simulink model "two_turtlebot3_waffle_pi_modelbaseMRAC2020"  (R2020b)
settings: Solver=VariableStepAuto  StartTime=0.0  StopTime=50  FixedStep=0.0001  RelTol=1e-3
values from neighbouring files (symbols this model uses):
  m = 5    [Traj.mat]    (also in dynamic_model.m = mc+2*mw; eightshape.mat)
  w = 0.015    [Assy_StateFlow_DataFile.m]    (also in eightshape.mat)
undefined symbols (not defined in the file or in its folder): X, Y, Z
libraries: sm_lib x258, nesl_utility x21, simulink x2, robotcorelib x2
(part 5 of 5)

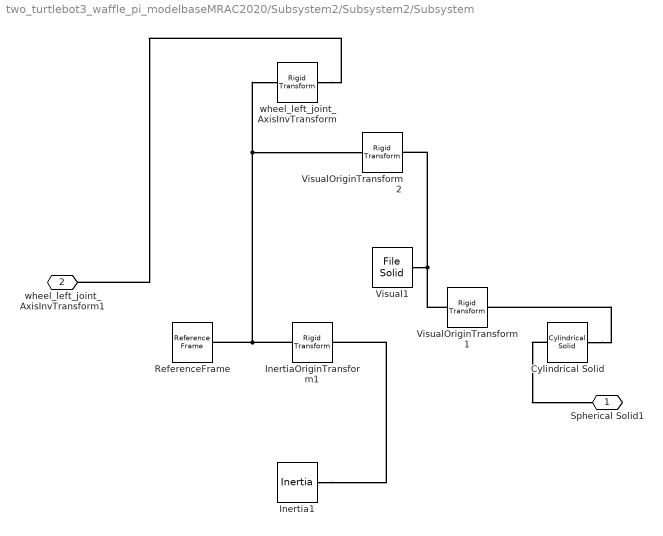
== system two_turtlebot3_waffle_pi_modelbaseMRAC2020/Subsystem2/Subsystem2/Subsystem ==
  Cylindrical Solid : sm_lib/Body Elements/Cylindrical Solid  GraphicAmbientColor=[0.15 0.15 0.15 1.0]  BasedOnType=Density  CenterOfMass=[0 0 0]  CenterOfMassUnits=m  GraphicDiffuseColor=[0.5 0.5 0.5]  CylinderLength=0.01  CylinderLengthUnits=m  CylinderRadius=0.033  CylinderRadiusUnits=m  Density=1000  DensityUnits=kg/m^3  DoExposeReferenceFrame=on  GraphicEmissiveColor=[0.0 0.0 0.0 1.0]  ExportEntireGeometry=on  SerializedFrames=<Frames/>  MarkerShape=Sphere  MarkerSize=10  GraphicType=FromGeometry  InertiaType=PointMass  Mass=0  MassUnits=kg  MomentsOfInertia=[1 1 1]  MomentsOfInertiaUnits=kg*m^2  GraphicOpacity=1.0  ProductsOfInertia=[0 0 0]  ProductsOfInertiaUnits=kg*m^2  GraphicShininess=75  GraphicSpecularColor=[0.5 0.5 0.5 1.0]  GraphicVisPropType=SimpleVisualProperties
  Inertia1 : sm_lib/Body Elements/Inertia  InertiaType=Custom  Mass=0.02849894  MassUnits=kg  CenterOfMass=[0, 0, 0]  CenterOfMassUnits=m  MomentsOfInertia=[1.117558e-05, 1.1192413e-05, 2.0712558e-05]  MomentsOfInertiaUnits=kg*m^2  ProductsOfInertia=[-1.4400107e-11, -5.9381719e-09, -4.2369783e-11]  ProductsOfInertiaUnits=kg*m^2  GraphicType=None  MarkerShape=Inertia  MarkerSize=20  GraphicVisPropType=SimpleVisualProperties  GraphicDiffuseColor=[0.5 0.5 0.5]  GraphicSpecularColor=[0.5 0.5 0.5 1.0]  GraphicAmbientColor=[0.15 0.15 0.15 1.0]  GraphicEmissiveColor=[0.0 0.0 0.0 1.0]  GraphicShininess=75  GraphicOpacity=1.0
  InertiaOriginTransform1 : sm_lib/Frames and Transforms/Rigid Transform  TranslationMethod=Cartesian  TranslationStandardOffset=0  TranslationLengthUnit=m  TranslationStandardAxis=+Z  TranslationCartesianOffset=[0, 0, 0]  TranslationROffset=0  TranslationROffsetUnits=m  TranslationZOffset=0  TranslationZOffsetUnits=m  TranslationThetaOffset=0  TranslationThetaOffsetUnits=deg  RotationMethod=RotationSequence  RotationAngleUnits=deg  RotationStandardAxis=+Z  RotationAngle=0.0  RotationArbitraryAxis=[0 0 1]  FollAlignAxisA=+X  BaseAlignAxisA=+Y  FollAlignAxisB=+Y  BaseAlignAxisB=+Z  RotationSequenceAxes=BaseAxes  RotationSequence=XYZ  RotationSequenceAngles=[0, 0, 0]  RotationSequenceAnglesUnits=rad  RotationMatrix=[1 0 0; 0 1 0; 0 0 1]
  ReferenceFrame : sm_lib/Frames and Transforms/Reference Frame
  Visual1 : sm_lib/Body Elements/File Solid  ExtGeomFileName=C:\Users\suyao\Desktop\tethered robot planning\simulation\Stateflow_Lab\CAD\right_tire.stl  UnitType=Custom  ExtGeomFileUnits=mm  StepReaderType=HEX  ExportConvexHullGeometry=on  InertiaType=Custom  Mass=0  MassUnits=kg  CenterOfMass=[0, 0, 0]  CenterOfMassUnits=m  MomentsOfInertia=[0, 0, 0]  MomentsOfInertiaUnits=kg*m^2  ProductsOfInertia=[0, 0, 0]  ProductsOfInertiaUnits=kg*m^2  BasedOnType=DensityFromFile  Density=1000  DensityUnits=kg/m^3  DoExposeReferenceFrame=on  SerializedFrames=<Frames/>  GraphicType=FromGeometry  MarkerShape=Sphere  MarkerSize=10  GraphicVisPropType=SimpleVisualProperties  GraphicDiffuseColor=[0.5, 0.5, 0.5]  GraphicSpecularColor=[0.5 0.5 0.5 1.0]  GraphicAmbientColor=[0.15 0.15 0.15 1.0]  GraphicEmissiveColor=[0.0 0.0 0.0 1.0]  GraphicShininess=75  GraphicOpacity=1
  VisualOriginTransform1 : sm_lib/Frames and Transforms/Rigid Transform  TranslationMethod=Cartesian  TranslationStandardOffset=0  TranslationLengthUnit=m  TranslationStandardAxis=+Z  TranslationCartesianOffset=[0, 0, 0]  TranslationROffset=0  TranslationROffsetUnits=m  TranslationZOffset=0  TranslationZOffsetUnits=m  TranslationThetaOffset=0  TranslationThetaOffsetUnits=deg  RotationMethod=StandardAxis  RotationAngleUnits=deg  RotationStandardAxis=+X  RotationAngle=90  RotationArbitraryAxis=[0 0 1]  FollAlignAxisA=+X  BaseAlignAxisA=+Y  FollAlignAxisB=+Y  BaseAlignAxisB=+Z  RotationSequenceAxes=BaseAxes  RotationSequence=XYZ  RotationSequenceAngles=[1.57, 0, 0]  RotationSequenceAnglesUnits=rad  RotationMatrix=[1 0 0; 0 1 0; 0 0 1]
  VisualOriginTransform2 : sm_lib/Frames and Transforms/Rigid Transform  TranslationMethod=Cartesian  TranslationStandardOffset=0  TranslationLengthUnit=m  TranslationStandardAxis=+Z  TranslationCartesianOffset=[0, 0, 0]  TranslationROffset=0  TranslationROffsetUnits=m  TranslationZOffset=0  TranslationZOffsetUnits=m  TranslationThetaOffset=0  TranslationThetaOffsetUnits=deg  RotationMethod=RotationSequence  RotationAngleUnits=deg  RotationStandardAxis=+Z  RotationAngle=0.0  RotationArbitraryAxis=[0 0 1]  FollAlignAxisA=+X  BaseAlignAxisA=+Y  FollAlignAxisB=+Y  BaseAlignAxisB=+Z  RotationSequenceAxes=BaseAxes  RotationSequence=XYZ  RotationSequenceAngles=[1.57, 0, 0]  RotationSequenceAnglesUnits=rad  RotationMatrix=[1 0 0; 0 1 0; 0 0 1]
  wheel_left_joint_AxisInvTransform : sm_lib/Frames and Transforms/Rigid Transform  TranslationMethod=Cartesian  TranslationStandardOffset=0  TranslationLengthUnit=m  TranslationStandardAxis=+Z  TranslationCartesianOffset=[0, 0, 0]  TranslationROffset=0  TranslationROffsetUnits=m  TranslationZOffset=0  TranslationZOffsetUnits=m  TranslationThetaOffset=0  TranslationThetaOffsetUnits=deg  RotationMethod=ArbitraryAxis  RotationAngleUnits=rad  RotationStandardAxis=+Z  RotationAngle=0  RotationArbitraryAxis=[1, 0, 0]  FollAlignAxisA=+X  BaseAlignAxisA=+Y  FollAlignAxisB=+Y  BaseAlignAxisB=+Z  RotationSequenceAxes=FollowerAxes  RotationSequence=XYX  RotationSequenceAngles=[0 0 0]  RotationSequenceAnglesUnits=deg  RotationMatrix=[1 0 0; 0 1 0; 0 0 1]
  Spherical Solid1 : PMIOPort  Side=Left
  wheel_left_joint_AxisInvTransform1 : PMIOPort  Port=2  Side=Right
  connections:
  wheel_left_joint_AxisInvTransform/RConn1 -- wheel_left_joint_AxisInvTransform1/RConn1
  ReferenceFrame/RConn1 -- InertiaOriginTransform1/LConn1 -- VisualOriginTransform2/LConn1 -- wheel_left_joint_AxisInvTransform/LConn1
  Visual1/RConn1 -- VisualOriginTransform1/LConn1 -- VisualOriginTransform2/RConn1
  Inertia1/RConn1 -- InertiaOriginTransform1/RConn1
  Cylindrical Solid/RConn1 -- VisualOriginTransform1/RConn1
  Cylindrical Solid/LConn1 -- Spherical Solid1/RConn1

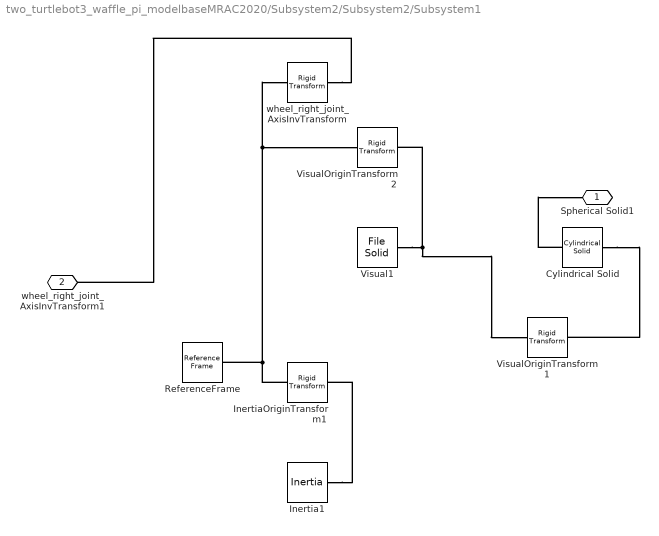
== system two_turtlebot3_waffle_pi_modelbaseMRAC2020/Subsystem2/Subsystem2/Subsystem1 ==
  Cylindrical Solid : sm_lib/Body Elements/Cylindrical Solid  GraphicAmbientColor=[0.15 0.15 0.15 1.0]  BasedOnType=Density  CenterOfMass=[0 0 0]  CenterOfMassUnits=m  GraphicDiffuseColor=[0.5 0.5 0.5]  CylinderLength=0.01  CylinderLengthUnits=m  CylinderRadius=0.032  CylinderRadiusUnits=m  Density=1000  DensityUnits=kg/m^3  DoExposeReferenceFrame=on  GraphicEmissiveColor=[0.0 0.0 0.0 1.0]  ExportEntireGeometry=on  SerializedFrames=<Frames/>  MarkerShape=Sphere  MarkerSize=10  GraphicType=FromGeometry  InertiaType=CalculateFromGeometry  Mass=1  MassUnits=kg  MomentsOfInertia=[1 1 1]  MomentsOfInertiaUnits=kg*m^2  GraphicOpacity=1.0  ProductsOfInertia=[0 0 0]  ProductsOfInertiaUnits=kg*m^2  GraphicShininess=75  GraphicSpecularColor=[0.5 0.5 0.5 1.0]  GraphicVisPropType=SimpleVisualProperties
  Inertia1 : sm_lib/Body Elements/Inertia  InertiaType=Custom  Mass=0.02849894  MassUnits=kg  CenterOfMass=[0, 0, 0]  CenterOfMassUnits=m  MomentsOfInertia=[1.117558e-05, 1.1192413e-05, 2.0712558e-05]  MomentsOfInertiaUnits=kg*m^2  ProductsOfInertia=[-1.4400107e-11, -5.9381719e-09, -4.2369783e-11]  ProductsOfInertiaUnits=kg*m^2  GraphicType=None  MarkerShape=Inertia  MarkerSize=20  GraphicVisPropType=SimpleVisualProperties  GraphicDiffuseColor=[0.5 0.5 0.5]  GraphicSpecularColor=[0.5 0.5 0.5 1.0]  GraphicAmbientColor=[0.15 0.15 0.15 1.0]  GraphicEmissiveColor=[0.0 0.0 0.0 1.0]  GraphicShininess=75  GraphicOpacity=1.0
  InertiaOriginTransform1 : sm_lib/Frames and Transforms/Rigid Transform  TranslationMethod=Cartesian  TranslationStandardOffset=0  TranslationLengthUnit=m  TranslationStandardAxis=+Z  TranslationCartesianOffset=[0, 0, 0]  TranslationROffset=0  TranslationROffsetUnits=m  TranslationZOffset=0  TranslationZOffsetUnits=m  TranslationThetaOffset=0  TranslationThetaOffsetUnits=deg  RotationMethod=RotationSequence  RotationAngleUnits=deg  RotationStandardAxis=+Z  RotationAngle=0.0  RotationArbitraryAxis=[0 0 1]  FollAlignAxisA=+X  BaseAlignAxisA=+Y  FollAlignAxisB=+Y  BaseAlignAxisB=+Z  RotationSequenceAxes=BaseAxes  RotationSequence=XYZ  RotationSequenceAngles=[0, 0, 0]  RotationSequenceAnglesUnits=rad  RotationMatrix=[1 0 0; 0 1 0; 0 0 1]
  ReferenceFrame : sm_lib/Frames and Transforms/Reference Frame
  Visual1 : sm_lib/Body Elements/File Solid  ExtGeomFileName=C:\Users\suyao\Desktop\tethered robot planning\simulation\Stateflow_Lab\CAD\right_tire.stl  UnitType=Custom  ExtGeomFileUnits=mm  StepReaderType=HEX  ExportConvexHullGeometry=on  InertiaType=Custom  Mass=0  MassUnits=kg  CenterOfMass=[0, 0, 0]  CenterOfMassUnits=m  MomentsOfInertia=[0, 0, 0]  MomentsOfInertiaUnits=kg*m^2  ProductsOfInertia=[0, 0, 0]  ProductsOfInertiaUnits=kg*m^2  BasedOnType=DensityFromFile  Density=1000  DensityUnits=kg/m^3  DoExposeReferenceFrame=on  SerializedFrames=<Frames/>  GraphicType=FromGeometry  MarkerShape=Sphere  MarkerSize=10  GraphicVisPropType=SimpleVisualProperties  GraphicDiffuseColor=[0.5, 0.5, 0.5]  GraphicSpecularColor=[0.5 0.5 0.5 1.0]  GraphicAmbientColor=[0.15 0.15 0.15 1.0]  GraphicEmissiveColor=[0.0 0.0 0.0 1.0]  GraphicShininess=75  GraphicOpacity=1
  VisualOriginTransform1 : sm_lib/Frames and Transforms/Rigid Transform  TranslationMethod=Cartesian  TranslationStandardOffset=0  TranslationLengthUnit=m  TranslationStandardAxis=+Z  TranslationCartesianOffset=[0, 0, 0]  TranslationROffset=0  TranslationROffsetUnits=m  TranslationZOffset=0  TranslationZOffsetUnits=m  TranslationThetaOffset=0  TranslationThetaOffsetUnits=deg  RotationMethod=StandardAxis  RotationAngleUnits=deg  RotationStandardAxis=+X  RotationAngle=90  RotationArbitraryAxis=[0 0 1]  FollAlignAxisA=+X  BaseAlignAxisA=+Y  FollAlignAxisB=+Y  BaseAlignAxisB=+Z  RotationSequenceAxes=BaseAxes  RotationSequence=XYZ  RotationSequenceAngles=[1.57, 0, 0]  RotationSequenceAnglesUnits=rad  RotationMatrix=[1 0 0; 0 1 0; 0 0 1]
  VisualOriginTransform2 : sm_lib/Frames and Transforms/Rigid Transform  TranslationMethod=Cartesian  TranslationStandardOffset=0  TranslationLengthUnit=m  TranslationStandardAxis=+Z  TranslationCartesianOffset=[0, 0, 0]  TranslationROffset=0  TranslationROffsetUnits=m  TranslationZOffset=0  TranslationZOffsetUnits=m  TranslationThetaOffset=0  TranslationThetaOffsetUnits=deg  RotationMethod=RotationSequence  RotationAngleUnits=deg  RotationStandardAxis=+Z  RotationAngle=0.0  RotationArbitraryAxis=[0 0 1]  FollAlignAxisA=+X  BaseAlignAxisA=+Y  FollAlignAxisB=+Y  BaseAlignAxisB=+Z  RotationSequenceAxes=BaseAxes  RotationSequence=XYZ  RotationSequenceAngles=[1.57, 0, 0]  RotationSequenceAnglesUnits=rad  RotationMatrix=[1 0 0; 0 1 0; 0 0 1]
  wheel_right_joint_AxisInvTransform : sm_lib/Frames and Transforms/Rigid Transform  TranslationMethod=Cartesian  TranslationStandardOffset=0  TranslationLengthUnit=m  TranslationStandardAxis=+Z  TranslationCartesianOffset=[0, 0, 0]  TranslationROffset=0  TranslationROffsetUnits=m  TranslationZOffset=0  TranslationZOffsetUnits=m  TranslationThetaOffset=0  TranslationThetaOffsetUnits=deg  RotationMethod=ArbitraryAxis  RotationAngleUnits=rad  RotationStandardAxis=+Z  RotationAngle=0  RotationArbitraryAxis=[1, 0, 0]  FollAlignAxisA=+X  BaseAlignAxisA=+Y  FollAlignAxisB=+Y  BaseAlignAxisB=+Z  RotationSequenceAxes=FollowerAxes  RotationSequence=XYX  RotationSequenceAngles=[0 0 0]  RotationSequenceAnglesUnits=deg  RotationMatrix=[1 0 0; 0 1 0; 0 0 1]
  Spherical Solid1 : PMIOPort  Side=Left
  wheel_right_joint_AxisInvTransform1 : PMIOPort  Port=2  Side=Right
  connections:
  Inertia1/RConn1 -- InertiaOriginTransform1/RConn1
  ReferenceFrame/RConn1 -- InertiaOriginTransform1/LConn1 -- VisualOriginTransform2/LConn1 -- wheel_right_joint_AxisInvTransform/LConn1
  Visual1/RConn1 -- VisualOriginTransform2/RConn1 -- VisualOriginTransform1/LConn1
  wheel_right_joint_AxisInvTransform/RConn1 -- wheel_right_joint_AxisInvTransform1/RConn1
  Cylindrical Solid/RConn1 -- VisualOriginTransform1/RConn1
  Cylindrical Solid/LConn1 -- Spherical Solid1/RConn1

== system two_turtlebot3_waffle_pi_modelbaseMRAC2020/Subsystem2/Subsystem2/Subsystem2 ==
  In1 : Inport
  PS-Simulink Converter : nesl_utility/PS-Simulink Converter  PhysicalDomain=network_engine_domain  SubClassName=ps_output  LeftPortType=input  RightPortType=output  PseudoPeriodic=off  Frequencies=[]  Unit=inherit  AffineConversion=off
      settings: SourceProductBaseCode=PW,SS
  Simulink-PS Converter : nesl_utility/Simulink-PS Converter  PhysicalDomain=network_engine_domain  SubClassName=ps_input  LeftPortType=input  RightPortType=output  PseudoPeriodic=off  Frequencies=[]  NoiseDistribution=none  NoiseParameters=[]  Unit=1  AffineConversion=off  FilteringAndDerivatives=provide  SimscapeFilterOrder=1  InputFilterTimeConstant=0.001  UdotUserProvided=0
      settings: SourceProductBaseCode=PW,SS
  wheel_right_joint : sm_lib/Joints/Revolute Joint  JointMode=Normal  SenseConstraintForce=off  SenseConstraintForceX=off  SenseConstraintForceY=off  SenseConstraintForceZ=off  SenseConstraintTorque=off  SenseConstraintTorqueX=off  SenseConstraintTorqueY=off  SenseConstraintTorqueZ=off  SenseTotalForce=off  SenseTotalForceX=off  SenseTotalForceY=off  SenseTotalForceZ=off  SenseTotalTorque=off  SenseTotalTorqueX=off  SenseTotalTorqueY=off  SenseTotalTorqueZ=off  CompositeWrenchDir=FollowerOnBase  CompositeWrenchFrame=BaseFrame  EquilibriumPosition=0  EquilibriumPositionUnits=deg  SpringStiffness=0  SpringStiffnessUnits=N*m/deg  DampingCoefficient=0  DampingCoefficientUnits=m^2*kg/s/rad  TorqueActuationMode=InputTorque  MotionActuationMode=ComputedMotion  SensePosition=off  SenseVelocity=on  SenseAcceleration=off  SenseTorqueForce=off  SenseLowerLimitTorqueForce=off  SenseUpperLimitTorqueForce=off  LowerLimitSpecify=off  LowerLimitBound=-90  LowerLimitBoundUnits=deg  LowerLimitStiffness=1e4  LowerLimitStiffnessUnits=N*m/deg  LowerLimitDamping=10  LowerLimitDampingUnits=N*m/(deg/s)  LowerLimitTransitionRegionWidth=0.1  LowerLimitTransitionRegionWidthUnits=deg  UpperLimitSpecify=off  UpperLimitBound=90  UpperLimitBoundUnits=deg  UpperLimitStiffness=1e4  UpperLimitStiffnessUnits=N*m/deg  UpperLimitDamping=10  UpperLimitDampingUnits=N*m/(deg/s)  UpperLimitTransitionRegionWidth=0.1  UpperLimitTransitionRegionWidthUnits=deg  PositionTargetSpecify=off  PositionTargetPriority=High  PositionTargetValue=0  PositionTargetValueUnits=deg  VelocityTargetSpecify=off  VelocityTargetPriority=High  VelocityTargetValue=0  VelocityTargetValueUnits=deg/s
  wheel_right_joint_AxisTransform : sm_lib/Frames and Transforms/Rigid Transform  TranslationMethod=Cartesian  TranslationStandardOffset=0  TranslationLengthUnit=m  TranslationStandardAxis=+Z  TranslationCartesianOffset=[0, 0, 0]  TranslationROffset=0  TranslationROffsetUnits=m  TranslationZOffset=0  TranslationZOffsetUnits=m  TranslationThetaOffset=0  TranslationThetaOffsetUnits=deg  RotationMethod=ArbitraryAxis  RotationAngleUnits=rad  RotationStandardAxis=+Z  RotationAngle=0  RotationArbitraryAxis=[1, 0, 0]  FollAlignAxisA=+X  BaseAlignAxisA=+Y  FollAlignAxisB=+Y  BaseAlignAxisB=+Z  RotationSequenceAxes=FollowerAxes  RotationSequence=XYX  RotationSequenceAngles=[0 0 0]  RotationSequenceAnglesUnits=deg  RotationMatrix=[1 0 0; 0 1 0; 0 0 1]
  wheel_right_joint_OriginTransform : sm_lib/Frames and Transforms/Rigid Transform  TranslationMethod=Cartesian  TranslationStandardOffset=0  TranslationLengthUnit=m  TranslationStandardAxis=+Z  TranslationCartesianOffset=[0, -0.144, 0.023]  TranslationROffset=0  TranslationROffsetUnits=m  TranslationZOffset=0  TranslationZOffsetUnits=m  TranslationThetaOffset=0  TranslationThetaOffsetUnits=deg  RotationMethod=RotationSequence  RotationAngleUnits=deg  RotationStandardAxis=+Z  RotationAngle=0.0  RotationArbitraryAxis=[0 0 1]  FollAlignAxisA=+X  BaseAlignAxisA=+Y  FollAlignAxisB=+Y  BaseAlignAxisB=+Z  RotationSequenceAxes=BaseAxes  RotationSequence=XYZ  RotationSequenceAngles=[-1.57, 0, 0]  RotationSequenceAnglesUnits=rad  RotationMatrix=[1 0 0; 0 1 0; 0 0 1]
  wheel_right_joint1 : PMIOPort  Side=Right
  wheel_right_joint_OriginTransform1 : PMIOPort  Port=2  Side=Left
  wires:
  In1/1 -> Simulink-PS Converter/1
  connections:
  wheel_right_joint_AxisTransform/RConn1 -- wheel_right_joint/LConn1
  wheel_right_joint_OriginTransform/LConn1 -- wheel_right_joint_OriginTransform1/RConn1
  wheel_right_joint/LConn2 -- Simulink-PS Converter/RConn1
  wheel_right_joint_AxisTransform/LConn1 -- wheel_right_joint_OriginTransform/RConn1
  wheel_right_joint1/RConn1 -- wheel_right_joint/RConn1
  wheel_right_joint/RConn2 -- PS-Simulink Converter/LConn1

== system two_turtlebot3_waffle_pi_modelbaseMRAC2020/Subsystem2/Subsystem2/Subsystem3 ==
  In1 : Inport
  PS-Simulink Converter1 : nesl_utility/PS-Simulink Converter  PhysicalDomain=network_engine_domain  SubClassName=ps_output  LeftPortType=input  RightPortType=output  PseudoPeriodic=off  Frequencies=[]  Unit=inherit  AffineConversion=off
      settings: SourceProductBaseCode=PW,SS
  Scope : Scope  NumInputPorts=2
  Simulink-PS Converter1 : nesl_utility/Simulink-PS Converter  PhysicalDomain=network_engine_domain  SubClassName=ps_input  LeftPortType=input  RightPortType=output  PseudoPeriodic=off  Frequencies=[]  NoiseDistribution=none  NoiseParameters=[]  Unit=1  AffineConversion=off  FilteringAndDerivatives=provide  SimscapeFilterOrder=1  InputFilterTimeConstant=0.001  UdotUserProvided=0
      settings: SourceProductBaseCode=PW,SS
  wheel_left_joint : sm_lib/Joints/Revolute Joint  JointMode=Normal  SenseConstraintForce=off  SenseConstraintForceX=off  SenseConstraintForceY=off  SenseConstraintForceZ=off  SenseConstraintTorque=off  SenseConstraintTorqueX=off  SenseConstraintTorqueY=off  SenseConstraintTorqueZ=off  SenseTotalForce=off  SenseTotalForceX=off  SenseTotalForceY=off  SenseTotalForceZ=off  SenseTotalTorque=off  SenseTotalTorqueX=off  SenseTotalTorqueY=off  SenseTotalTorqueZ=off  CompositeWrenchDir=FollowerOnBase  CompositeWrenchFrame=BaseFrame  EquilibriumPosition=0  EquilibriumPositionUnits=deg  SpringStiffness=0  SpringStiffnessUnits=N*m/deg  DampingCoefficient=0  DampingCoefficientUnits=m^2*kg/s/rad  TorqueActuationMode=InputTorque  MotionActuationMode=ComputedMotion  SensePosition=off  SenseVelocity=on  SenseAcceleration=off  SenseTorqueForce=off  SenseLowerLimitTorqueForce=off  SenseUpperLimitTorqueForce=off  LowerLimitSpecify=off  LowerLimitBound=-90  LowerLimitBoundUnits=deg  LowerLimitStiffness=1e4  LowerLimitStiffnessUnits=N*m/deg  LowerLimitDamping=10  LowerLimitDampingUnits=N*m/(deg/s)  LowerLimitTransitionRegionWidth=0.1  LowerLimitTransitionRegionWidthUnits=deg  UpperLimitSpecify=off  UpperLimitBound=90  UpperLimitBoundUnits=deg  UpperLimitStiffness=1e4  UpperLimitStiffnessUnits=N*m/deg  UpperLimitDamping=10  UpperLimitDampingUnits=N*m/(deg/s)  UpperLimitTransitionRegionWidth=0.1  UpperLimitTransitionRegionWidthUnits=deg  PositionTargetSpecify=off  PositionTargetPriority=High  PositionTargetValue=0  PositionTargetValueUnits=deg  VelocityTargetSpecify=off  VelocityTargetPriority=High  VelocityTargetValue=0  VelocityTargetValueUnits=deg/s
  wheel_left_joint_AxisTransform : sm_lib/Frames and Transforms/Rigid Transform  TranslationMethod=Cartesian  TranslationStandardOffset=0  TranslationLengthUnit=m  TranslationStandardAxis=+Z  TranslationCartesianOffset=[0, 0, 0]  TranslationROffset=0  TranslationROffsetUnits=m  TranslationZOffset=0  TranslationZOffsetUnits=m  TranslationThetaOffset=0  TranslationThetaOffsetUnits=deg  RotationMethod=ArbitraryAxis  RotationAngleUnits=rad  RotationStandardAxis=+Z  RotationAngle=0  RotationArbitraryAxis=[1, 0, 0]  FollAlignAxisA=+X  BaseAlignAxisA=+Y  FollAlignAxisB=+Y  BaseAlignAxisB=+Z  RotationSequenceAxes=FollowerAxes  RotationSequence=XYX  RotationSequenceAngles=[0 0 0]  RotationSequenceAnglesUnits=deg  RotationMatrix=[1 0 0; 0 1 0; 0 0 1]
  wheel_left_joint_OriginTransform : sm_lib/Frames and Transforms/Rigid Transform  TranslationMethod=Cartesian  TranslationStandardOffset=0  TranslationLengthUnit=m  TranslationStandardAxis=+Z  TranslationCartesianOffset=[0, 0.144, 0.023]  TranslationROffset=0  TranslationROffsetUnits=m  TranslationZOffset=0  TranslationZOffsetUnits=m  TranslationThetaOffset=0  TranslationThetaOffsetUnits=deg  RotationMethod=RotationSequence  RotationAngleUnits=deg  RotationStandardAxis=+Z  RotationAngle=0.0  RotationArbitraryAxis=[0 0 1]  FollAlignAxisA=+X  BaseAlignAxisA=+Y  FollAlignAxisB=+Y  BaseAlignAxisB=+Z  RotationSequenceAxes=BaseAxes  RotationSequence=XYZ  RotationSequenceAngles=[-1.57, 0, 0]  RotationSequenceAnglesUnits=rad  RotationMatrix=[1 0 0; 0 1 0; 0 0 1]
  wheel_left_joint1 : PMIOPort  Side=Right
  wheel_left_joint_OriginTransform1 : PMIOPort  Port=2  Side=Left
  wires:
  PS-Simulink Converter1/1 -> Scope/2
  In1/1 -> Simulink-PS Converter1/1
  connections:
  wheel_left_joint_OriginTransform/LConn1 -- wheel_left_joint_OriginTransform1/RConn1
  wheel_left_joint_AxisTransform/LConn1 -- wheel_left_joint_OriginTransform/RConn1
  wheel_left_joint/LConn2 -- Simulink-PS Converter1/RConn1
  wheel_left_joint_AxisTransform/RConn1 -- wheel_left_joint/LConn1
  PS-Simulink Converter1/LConn1 -- wheel_left_joint/RConn2
  wheel_left_joint1/RConn1 -- wheel_left_joint/RConn1

== matlab function two_turtlebot3_waffle_pi_modelbaseMRAC2020/Subsystem/MATLAB Function1 ==
  data: X input; V output; X_dot input; X_r input
function V  = fcn(X,X_dot,X_r)
   err_x=X(1)-X_r(1);
   err_y=X(2)-X_r(2);
   phi=X_r(3); d=0.288; r=0.033;
   lx=2.0; ly=2.00; kx=5; ky=5;
   xx=X_dot(1)+lx*tanh(kx/lx*err_x);
   yy=X_dot(2)+ly*tanh(ky/ly*err_y);
   K=[cos(phi) sin(phi); -1/d*sin(phi) 1/d*cos(phi)];
   V=K*[xx;yy];
%    v=V(1); w=V(2);
%    A=[1/2 1/2; 1/d -1/d];
%    vv=(A^-1)*V;
%    vr=V(1)+d/2*V(2); vl=V(1)-d/2*V(2);
%    vr=vr/r; vl=vl/r;
end

== matlab function two_turtlebot3_waffle_pi_modelbaseMRAC2020/MATLAB Function ==
  data: t input; X1 output; X1_dot output; X2 output; X2_dot output; traj input; X1_old input; X2_old input; X1_old output; X2_old output
function [X1,X1_dot,X2,X2_dot,X1_old,X2_old] = fcn(t, traj,X1_old,X2_old)
dt=0.01;
i=floor(t/dt);
x1=traj(1); y1=traj(2);
x2=traj(3); y2=traj(4);
X1=[x1;y1]; X2=[x2;y2];
X1_dot=(X1-X1_old)/dt;
X2_dot=(X2-X2_old)/dt;
X1_old=X1;
X2_old=X2;

== matlab function two_turtlebot3_waffle_pi_modelbaseMRAC2020/Subsystem/MATLAB Function2 ==
  data: v input; v_dot input; Xr input; Xr_dot input; tau output; vr output; delta input; delta_r input; delta_dot output; deltar_dot output
function [tau,vr,delta_dot,deltar_dot] =fcn(v,v_dot,Xr,Xr_dot,delta,delta_r)
  t=Xr(3);  %v_dot=[0;0];
  x_d=Xr_dot(1); y_d=Xr_dot(2); t_dot=Xr_dot(3); 
  l=0.02;
  r=0.033; R=0.288; 
  m=1.42; J=0.0146;

  S=[cos(t) -l*sin(t); sin(t) l*cos(t); 0 1];
  vr=pinv(S)*Xr_dot;  %vr(2)=-vr(2); v(2)=-v(2);
  S_dot=[-sin(t)*t_dot -l*cos(t)*t_dot; cos(t)*t_dot -l*sin(t)*t_dot; 0 0];
  M=[m 0 m*l*sin(t);0 m -m*l*cos(t);m*l*sin(t) -m*l*cos(t) J];
  Vm=[0 0 m*l*t_dot*cos(t); 0 0 m*l*t_dot*sin(t); 0 0 0];
  E=1/r*[cos(t) cos(t); sin(t) sin(t); R -R];

  M_bar=S'*M*S;  V_bar=S'*M*S_dot+S'*Vm*S;
  E_bar=S'*E;  %
  tau=(E_bar^-1)*(M_bar*v_dot+V_bar*v);
  K=diag([10,4]); 
  P=[0.05,0;0,0.1]; a=20; b=-20;  
  e=v-vr; %e(2)=-e(2);
  ur=v_dot+K*v;
  uk=-K*vr+ur;
  ua=delta_r*ur-delta*vr;
  we=P*e;
  ubar=uk; %ua
  %ubar(2)=-ubar(2);
  u=ubar+(M_bar-eye(2))*v_dot+V_bar*v;  
  tau=(E_bar^-1)*u;
  delta_dot=-a*we*vr';
  deltar_dot=b*we*ur';
end

== matlab function two_turtlebot3_waffle_pi_modelbaseMRAC2020/Subsystem1/MATLAB Function1 ==
  data: X input; V output; X_dot input; X_r input
function V  = fcn(X,X_dot,X_r)
   err_x=X(1)-X_r(1);
   err_y=X(2)-X_r(2);
   phi=X_r(3); d=0.288; r=0.033;
   lx=2.0; ly=2.00; kx=5; ky=5;
   xx=X_dot(1)+lx*tanh(kx/lx*err_x);
   yy=X_dot(2)+ly*tanh(ky/ly*err_y);
   K=[cos(phi) sin(phi); -1/d*sin(phi) 1/d*cos(phi)];
   V=K*[xx;yy];
%    v=V(1); w=V(2);
%    A=[1/2 1/2; 1/d -1/d];
%    vv=(A^-1)*V;
%    vr=V(1)+d/2*V(2); vl=V(1)-d/2*V(2);
%    vr=vr/r; vl=vl/r;
end

== matlab function two_turtlebot3_waffle_pi_modelbaseMRAC2020/Subsystem1/MATLAB Function2 ==
  data: v input; v_dot input; Xr input; Xr_dot input; tau output; vr output; delta input; delta_r input; delta_dot output; deltar_dot output
function [tau,vr,delta_dot,deltar_dot] =fcn(v,v_dot,Xr,Xr_dot,delta,delta_r)
  t=Xr(3);  %v_dot=[0;0];
  x_d=Xr_dot(1); y_d=Xr_dot(2); t_dot=Xr_dot(3); 
  l=0.02;
  r=0.033; R=0.288; 
  m=1.42; J=0.0146;

  S=[cos(t) -l*sin(t); sin(t) l*cos(t); 0 1];
  vr=pinv(S)*Xr_dot;  %vr(2)=-vr(2); v(2)=-v(2);
  S_dot=[-sin(t)*t_dot -l*cos(t)*t_dot; cos(t)*t_dot -l*sin(t)*t_dot; 0 0];
  M=[m 0 m*l*sin(t);0 m -m*l*cos(t);m*l*sin(t) -m*l*cos(t) J];
  Vm=[0 0 m*l*t_dot*cos(t); 0 0 m*l*t_dot*sin(t); 0 0 0];
  E=1/r*[cos(t) cos(t); sin(t) sin(t); R -R];

  M_bar=S'*M*S;  V_bar=S'*M*S_dot+S'*Vm*S;
  E_bar=S'*E;  %
  tau=(E_bar^-1)*(M_bar*v_dot+V_bar*v);
  K=diag([10,4]); 
  P=[0.05,0;0,0.1]; a=20; b=-20;  
  e=v-vr; %e(2)=-e(2);
  ur=v_dot+K*v;
  uk=-K*vr+ur;
  ua=delta_r*ur-delta*vr;
  we=P*e;
  ubar=uk; %ua
  %ubar(2)=-ubar(2);
  u=ubar+(M_bar-eye(2))*v_dot+V_bar*v;  
  tau=(E_bar^-1)*u;
  delta_dot=-a*we*vr';
  deltar_dot=b*we*ur';
end
